simulink model "D_forward_dynamic_sim"  (R2017a)
settings: Solver=ode45  StartTime=0.0  StopTime=1  RelTol=1e-3  EnableMultiTasking=on
InitFcn:
  | ImportVars
settings Model: Creator=gwu  LastModifiedBy=Axel
settings DataIOCC: LimitDataPoints=on  SaveFormat=Array  SignalLoggingSaveFormat=ModelDataLogs
settings OptimizationCC: ExpressionDepthLimit=2147483647  LifeSpan=inf
settings DebuggingCC: UnderspecifiedInitializationDetection=Classic  MergeDetectMultiDrivingBlocksExec=none  SolverPrmCheckMsg=warning  FcnCallInpInsideContextMsg=warning  StateNameClashWarn=warning  SFUnexpectedBacktrackingDiag=warning  SFNoUnconditionalDefaultTransitionDiag=warning  SFExecutionAtInitializationDiag=none
settings HardwareCC: ProdBitPerPointer=32  ProdBitPerSizeT=32  ProdBitPerPtrDiffT=32  ProdLargestAtomicFloat=None  ProdIntDivRoundTo=Undefined  ProdEndianess=Unspecified  ProdWordSize=32  ProdHWDeviceType=32-bit Generic
settings ModelReferenceCC: PropagateSignalLabelsOutOfModel=off
settings RTWCC: TargetLang=C++
settings GRTTargetCC: TargetLangStandard=C89/C90 (ANSI)  GeneratePreprocessorConditionals=Disable all
settings ConfigComp: CovMetricSettings=dw  CovHtmlReporting=on  CovSaveCumulativeToWorkspaceVar=on  CovSaveSingleToWorkspaceVar=on  CovExternalEMLEnable=off

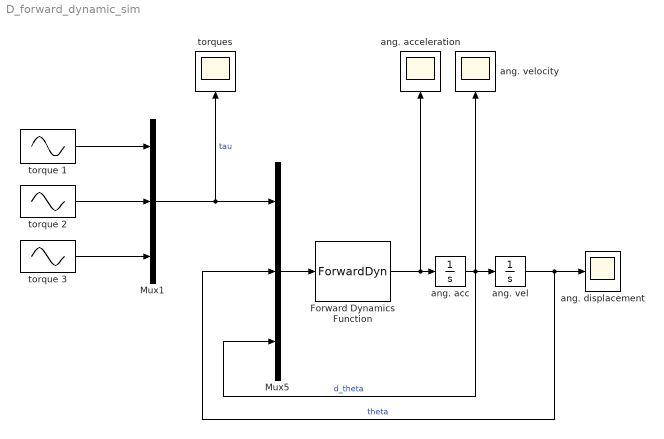
== system D_forward_dynamic_sim ==
  Forward Dynamics Function : MATLABFcn  MATLABFcn=ForwardDyn  OutputDimensions=3
  Mux1 : Mux  Inputs=3
  Mux5 : Mux  Inputs=3
  ang. acc : Integrator
  ang. acceleration : Scope
  ang. displacement : Scope
  ang. vel : Integrator
  ang. velocity : Scope
  torque 1 : Sin  Amplitude=0  Frequency=2  SampleTime=0
  torque 2 : Sin  Amplitude=1.4  Frequency=2  SampleTime=0
  torque 3 : Sin  Amplitude=0.397  Frequency=2  SampleTime=0
  torques : Scope
  wires:
  ang. acc/1 -> ang. vel/1, Mux5/3, ang. velocity/1  "d_theta"
  Forward Dynamics Function/1 -> ang. acc/1, ang. acceleration/1
  Mux5/1 -> Forward Dynamics Function/1
  torque 2/1 -> Mux1/2
  torque 1/1 -> Mux1/1
  Mux1/1 -> Mux5/1, torques/1  "tau"
  ang. vel/1 -> ang. displacement/1, Mux5/2  "theta"
  torque 3/1 -> Mux1/3
